simulink model "PID_Control"  (R2020b)
settings: Solver=VariableStepAuto  StartTime=0.0  StopTime=10.0  RelTol=1e-3
model mask{Kp=0, Ki=0, Kd=0}
model workspace (MAT data in the model file):
  Kd = 0
  Ki = 0
  Kp = 0
settings Model: DataDictionary=motor_speed_data.sldd  ParameterArgumentNames=Kd,Ki,Kp  OrderedModelArguments=off  Creator=Lenovo  LastModifiedBy=Lenovo
settings DataIOCC: SaveOutput=off  SaveTime=off

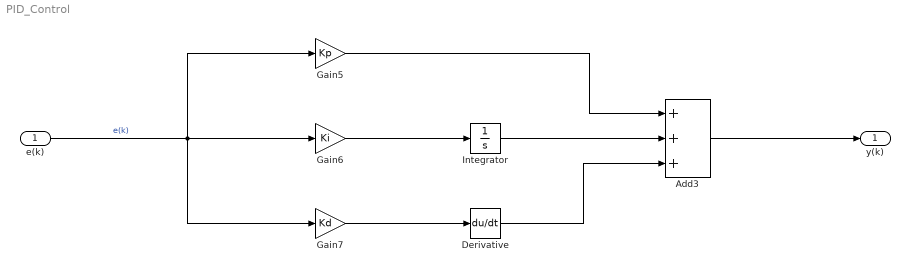
== system PID_Control ==
  e(k) : Inport  OutDataTypeStr=double  PortDimensions=1  SampleTime=0
  Add3 : Sum  Inputs=+++
  Derivative : Derivative
  Gain5 : Gain  Gain=Kp
  Gain6 : Gain  Gain=Ki
  Gain7 : Gain  Gain=Kd
  Integrator : Integrator
  y(k) : Outport  OutDataTypeStr=double  PortDimensions=1  SampleTime=0
  wires:
  e(k)/1 -> Gain7/1, Gain6/1, Gain5/1  "e(k)"
  Derivative/1 -> Add3/3
  Integrator/1 -> Add3/2
  Add3/1 -> y(k)/1
  Gain5/1 -> Add3/1
  Gain6/1 -> Integrator/1
  Gain7/1 -> Derivative/1
